simulink model "hbf_fft"  (R2015a)
settings: Solver=ode45  StartTime=0.0  StopTime=240300  RelTol=1e-3
model workspace (MAT data in the model file):
  MCOS : class17 (value not decoded)
  MCOS : class17 (value not decoded)
undefined symbols (not defined in the file or in its folder): a, b
libraries: xbsIndex_r4 x234, dspswit3 x1, commanapbnd3 x1, commseqgen2 x1, dspsigops x1
(part 2 of 2)

== system hbf_fft/nfftCounter/NegEdgeDet ==
  In1 : Inport
  Inverter : xbsIndex_r4/Inverter  en=off  latency=0  dbl_ovrd=off  block_type=inv
  Logical : xbsIndex_r4/Logical  logical_function=AND  inputs=2  en=off  latency=0  precision=Full  arith_type=Unsigned  n_bits=16  bin_pt=0  align_bp=on  dbl_ovrd=off  block_type=logical
  Register : xbsIndex_r4/Register  init=0  rst=off  en=off  dbl_ovrd=off  block_type=register
  Out1 : Outport
  wires:
  Register/1 -> Logical/1
  Inverter/1 -> Logical/2
  Logical/1 -> Out1/1
  In1/1 -> Inverter/1, Register/1

== system hbf_fft/nfftCounter/PosEdgeDet1 ==
  In1 : Inport
  Inverter : xbsIndex_r4/Inverter  en=off  latency=0  dbl_ovrd=off  block_type=inv
  Logical : xbsIndex_r4/Logical  logical_function=AND  inputs=2  en=off  latency=0  precision=Full  arith_type=Unsigned  n_bits=16  bin_pt=0  align_bp=on  dbl_ovrd=off  block_type=logical
  Register : xbsIndex_r4/Register  init=0  rst=off  en=off  dbl_ovrd=off  block_type=register
  Out1 : Outport
  wires:
  Logical/1 -> Out1/1
  In1/1 -> Logical/2, Register/1
  Register/1 -> Inverter/1
  Inverter/1 -> Logical/1

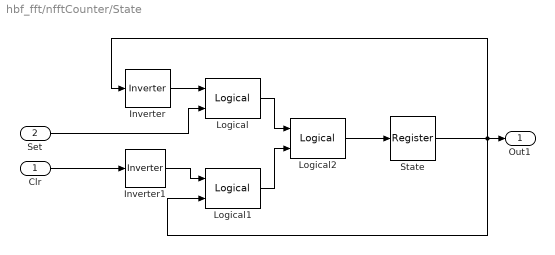
== system hbf_fft/nfftCounter/State ==
  Clr : Inport
  Set : Inport  Port=2
  Inverter : xbsIndex_r4/Inverter  en=off  latency=0  dbl_ovrd=off  block_type=inv
  Inverter1 : xbsIndex_r4/Inverter  en=off  latency=0  dbl_ovrd=off  block_type=inv
  Logical : xbsIndex_r4/Logical  logical_function=AND  inputs=2  en=off  latency=0  precision=Full  arith_type=Unsigned  n_bits=16  bin_pt=0  align_bp=on  dbl_ovrd=off  block_type=logical
  Logical1 : xbsIndex_r4/Logical  logical_function=AND  inputs=2  en=off  latency=0  precision=Full  arith_type=Unsigned  n_bits=16  bin_pt=0  align_bp=on  dbl_ovrd=off  block_type=logical
  Logical2 : xbsIndex_r4/Logical  logical_function=OR  inputs=2  en=off  latency=0  precision=Full  arith_type=Unsigned  n_bits=16  bin_pt=0  align_bp=on  dbl_ovrd=off  block_type=logical
  State : xbsIndex_r4/Register  init=0  rst=off  en=off  dbl_ovrd=off  block_type=register
  Out1 : Outport
  wires:
  Inverter1/1 -> Logical1/1
  Logical2/1 -> State/1
  Logical/1 -> Logical2/1
  Clr/1 -> Inverter1/1
  State/1 -> Out1/1, Logical1/2, Inverter/1
  Set/1 -> Logical/2
  Logical1/1 -> Logical2/2
  Inverter/1 -> Logical/1

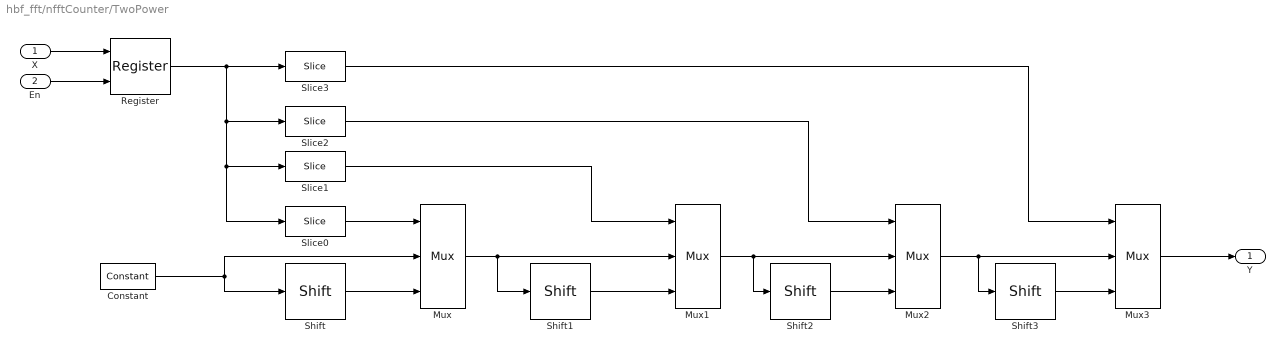
== system hbf_fft/nfftCounter/TwoPower ==
  X : Inport
  En : Inport  Port=2
  Constant : xbsIndex_r4/Constant  const=1.0  gui_display_data_type=Fixed-point  arith_type=Unsigned  n_bits=13  bin_pt=0  preci_type=Single  exp_width=8  frac_width=24  explicit_period=off  period=1  equ=P=C  opselect=C  inp2=PCIN>>17  opr=+  inp1=P  carry=CIN  dbl_ovrd=off  block_type=constant
  Mux : xbsIndex_r4/Mux  inputs=2  en=off  latency=0  precision=Full  arith_type=Unsigned  n_bits=16  bin_pt=14  quantization=Truncate  overflow=Wrap  dbl_ovrd=off  block_type=mux
  Mux1 : xbsIndex_r4/Mux  inputs=2  en=off  latency=0  precision=Full  arith_type=Unsigned  n_bits=16  bin_pt=14  quantization=Truncate  overflow=Wrap  dbl_ovrd=off  block_type=mux
  Mux2 : xbsIndex_r4/Mux  inputs=2  en=off  latency=0  precision=Full  arith_type=Unsigned  n_bits=16  bin_pt=14  quantization=Truncate  overflow=Wrap  dbl_ovrd=off  block_type=mux
  Mux3 : xbsIndex_r4/Mux  inputs=2  en=off  latency=1  precision=Full  arith_type=Unsigned  n_bits=16  bin_pt=14  quantization=Truncate  overflow=Wrap  dbl_ovrd=off  block_type=mux
  Register : xbsIndex_r4/Register  init=0  rst=off  en=on  dbl_ovrd=off  block_type=register
  Shift : xbsIndex_r4/Shift  shift_dir=Left  shift_bits=1  en=off  latency=0  precision=Full  arith_type="Signed  (2's comp)"  n_bits=16  bin_pt=14  quantization=Truncate  overflow=Wrap  dbl_ovrd=off  block_type=shift
  Shift1 : xbsIndex_r4/Shift  shift_dir=Left  shift_bits=2  en=off  latency=0  precision=Full  arith_type="Signed  (2's comp)"  n_bits=16  bin_pt=14  quantization=Truncate  overflow=Wrap  dbl_ovrd=off  block_type=shift
  Shift2 : xbsIndex_r4/Shift  shift_dir=Left  shift_bits=4  en=off  latency=0  precision=Full  arith_type="Signed  (2's comp)"  n_bits=16  bin_pt=14  quantization=Truncate  overflow=Wrap  dbl_ovrd=off  block_type=shift
  Shift3 : xbsIndex_r4/Shift  shift_dir=Left  shift_bits=8  en=off  latency=0  precision=Full  arith_type="Signed  (2's comp)"  n_bits=16  bin_pt=14  quantization=Truncate  overflow=Wrap  dbl_ovrd=off  block_type=shift
  Slice0 : xbsIndex_r4/Slice  nbits=1  boolean_output=off  mode=Lower Bit Location + Width  bit1=0  base1=MSB of Input  bit0=0  base0=LSB of Input  dbl_ovrd=off  block_type=slice
  Slice1 : xbsIndex_r4/Slice  nbits=1  boolean_output=off  mode=Lower Bit Location + Width  bit1=0  base1=MSB of Input  bit0=1  base0=LSB of Input  dbl_ovrd=off  block_type=slice
  Slice2 : xbsIndex_r4/Slice  nbits=1  boolean_output=off  mode=Lower Bit Location + Width  bit1=0  base1=MSB of Input  bit0=2  base0=LSB of Input  dbl_ovrd=off  block_type=slice
  Slice3 : xbsIndex_r4/Slice  nbits=1  boolean_output=off  mode=Lower Bit Location + Width  bit1=0  base1=MSB of Input  bit0=3  base0=LSB of Input  dbl_ovrd=off  block_type=slice
  Y : Outport
  wires:
  Constant/1 -> Shift/1, Mux/2
  X/1 -> Register/1
  Slice0/1 -> Mux/1
  Shift/1 -> Mux/3
  Slice1/1 -> Mux1/1
  Shift1/1 -> Mux1/3
  Slice2/1 -> Mux2/1
  Shift2/1 -> Mux2/3
  Slice3/1 -> Mux3/1
  Shift3/1 -> Mux3/3
  Mux/1 -> Shift1/1, Mux1/2
  Mux1/1 -> Shift2/1, Mux2/2
  Mux2/1 -> Shift3/1, Mux3/2
  Register/1 -> Slice0/1, Slice1/1, Slice2/1, Slice3/1
  En/1 -> Register/2
  Mux3/1 -> Y/1

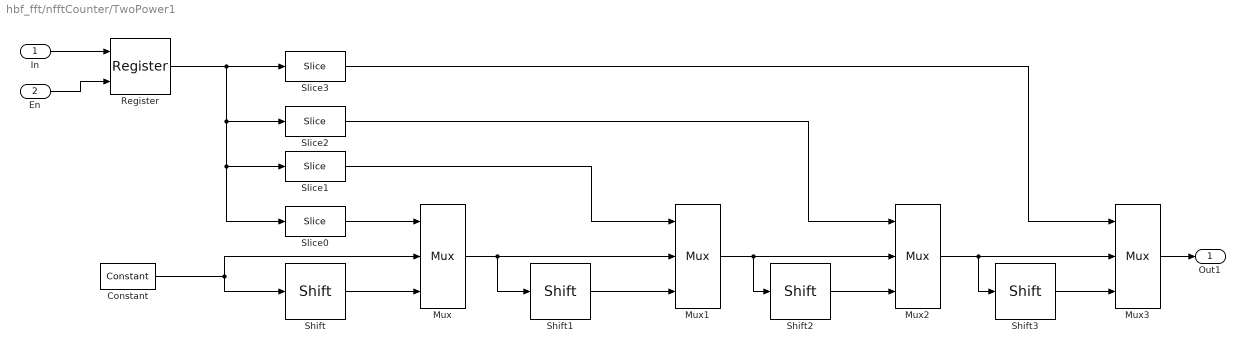
== system hbf_fft/nfftCounter/TwoPower1 ==
  In : Inport
  En : Inport  Port=2
  Constant : xbsIndex_r4/Constant  const=1.0  gui_display_data_type=Fixed-point  arith_type=Unsigned  n_bits=13  bin_pt=0  preci_type=Single  exp_width=8  frac_width=24  explicit_period=off  period=1  equ=P=C  opselect=C  inp2=PCIN>>17  opr=+  inp1=P  carry=CIN  dbl_ovrd=off  block_type=constant
  Mux : xbsIndex_r4/Mux  inputs=2  en=off  latency=0  precision=Full  arith_type=Unsigned  n_bits=16  bin_pt=14  quantization=Truncate  overflow=Wrap  dbl_ovrd=off  block_type=mux
  Mux1 : xbsIndex_r4/Mux  inputs=2  en=off  latency=0  precision=Full  arith_type=Unsigned  n_bits=16  bin_pt=14  quantization=Truncate  overflow=Wrap  dbl_ovrd=off  block_type=mux
  Mux2 : xbsIndex_r4/Mux  inputs=2  en=off  latency=0  precision=Full  arith_type=Unsigned  n_bits=16  bin_pt=14  quantization=Truncate  overflow=Wrap  dbl_ovrd=off  block_type=mux
  Mux3 : xbsIndex_r4/Mux  inputs=2  en=off  latency=1  precision=Full  arith_type=Unsigned  n_bits=16  bin_pt=14  quantization=Truncate  overflow=Wrap  dbl_ovrd=off  block_type=mux
  Register : xbsIndex_r4/Register  init=0  rst=off  en=on  dbl_ovrd=off  block_type=register
  Shift : xbsIndex_r4/Shift  shift_dir=Left  shift_bits=1  en=off  latency=0  precision=Full  arith_type="Signed  (2's comp)"  n_bits=16  bin_pt=14  quantization=Truncate  overflow=Wrap  dbl_ovrd=off  block_type=shift
  Shift1 : xbsIndex_r4/Shift  shift_dir=Left  shift_bits=2  en=off  latency=0  precision=Full  arith_type="Signed  (2's comp)"  n_bits=16  bin_pt=14  quantization=Truncate  overflow=Wrap  dbl_ovrd=off  block_type=shift
  Shift2 : xbsIndex_r4/Shift  shift_dir=Left  shift_bits=4  en=off  latency=0  precision=Full  arith_type="Signed  (2's comp)"  n_bits=16  bin_pt=14  quantization=Truncate  overflow=Wrap  dbl_ovrd=off  block_type=shift
  Shift3 : xbsIndex_r4/Shift  shift_dir=Left  shift_bits=8  en=off  latency=0  precision=Full  arith_type="Signed  (2's comp)"  n_bits=16  bin_pt=14  quantization=Truncate  overflow=Wrap  dbl_ovrd=off  block_type=shift
  Slice0 : xbsIndex_r4/Slice  nbits=1  boolean_output=off  mode=Lower Bit Location + Width  bit1=0  base1=MSB of Input  bit0=0  base0=LSB of Input  dbl_ovrd=off  block_type=slice
  Slice1 : xbsIndex_r4/Slice  nbits=1  boolean_output=off  mode=Lower Bit Location + Width  bit1=0  base1=MSB of Input  bit0=1  base0=LSB of Input  dbl_ovrd=off  block_type=slice
  Slice2 : xbsIndex_r4/Slice  nbits=1  boolean_output=off  mode=Lower Bit Location + Width  bit1=0  base1=MSB of Input  bit0=2  base0=LSB of Input  dbl_ovrd=off  block_type=slice
  Slice3 : xbsIndex_r4/Slice  nbits=1  boolean_output=off  mode=Lower Bit Location + Width  bit1=0  base1=MSB of Input  bit0=3  base0=LSB of Input  dbl_ovrd=off  block_type=slice
  Out1 : Outport
  wires:
  Constant/1 -> Shift/1, Mux/2
  In/1 -> Register/1
  Slice0/1 -> Mux/1
  Shift/1 -> Mux/3
  Slice1/1 -> Mux1/1
  Shift1/1 -> Mux1/3
  Slice2/1 -> Mux2/1
  Shift2/1 -> Mux2/3
  Slice3/1 -> Mux3/1
  Shift3/1 -> Mux3/3
  Mux/1 -> Shift1/1, Mux1/2
  Mux1/1 -> Shift2/1, Mux2/2
  Mux2/1 -> Shift3/1, Mux3/2
  Register/1 -> Slice0/1, Slice1/1, Slice2/1, Slice3/1
  En/1 -> Register/2
  Mux3/1 -> Out1/1

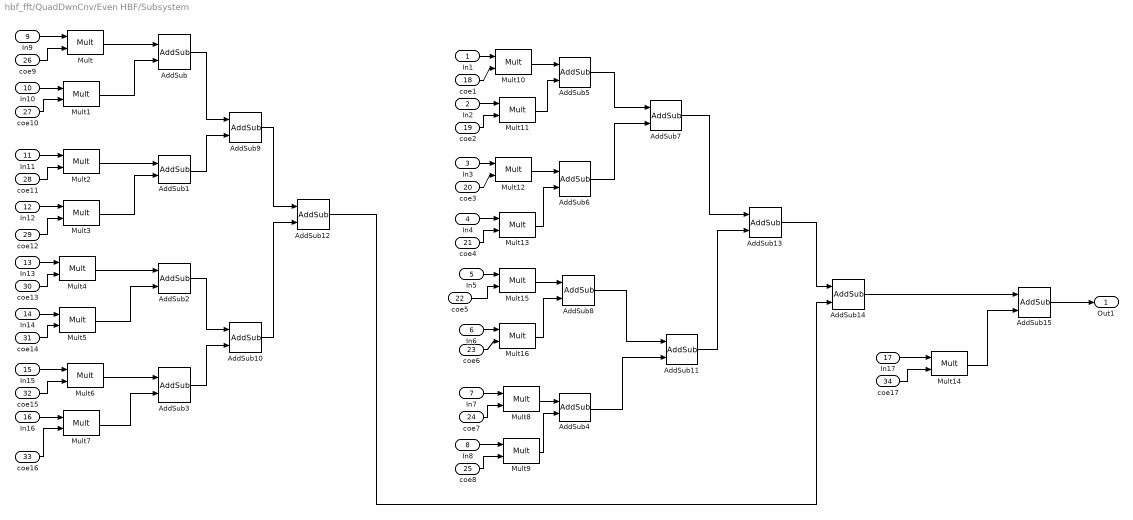
== system hbf_fft/QuadDwnCnv/Even HBF/Subsystem ==
  In1 : Inport
  In2 : Inport  Port=2
  In3 : Inport  Port=3
  In4 : Inport  Port=4
  In5 : Inport  Port=5
  In6 : Inport  Port=6
  In7 : Inport  Port=7
  In8 : Inport  Port=8
  In9 : Inport  Port=9
  In10 : Inport  Port=10
  In11 : Inport  Port=11
  In12 : Inport  Port=12
  In13 : Inport  Port=13
  In14 : Inport  Port=14
  In15 : Inport  Port=15
  In16 : Inport  Port=16
  In17 : Inport  Port=17
  coe1 : Inport  Port=18
  coe2 : Inport  Port=19
  coe3 : Inport  Port=20
  coe4 : Inport  Port=21
  coe5 : Inport  Port=22
  coe6 : Inport  Port=23
  coe7 : Inport  Port=24
  coe8 : Inport  Port=25
  coe9 : Inport  Port=26
  coe10 : Inport  Port=27
  coe11 : Inport  Port=28
  coe12 : Inport  Port=29
  coe13 : Inport  Port=30
  coe14 : Inport  Port=31
  coe15 : Inport  Port=32
  coe16 : Inport  Port=33
  coe17 : Inport  Port=34
  AddSub{,1..15} (16 alike) : xbsIndex_r4/AddSub  mode=Addition  use_carryin=off  use_carryout=off  en=off  latency=0  precision=Full  arith_type=Unsigned  n_bits=16  bin_pt=14  quantization=Truncate  overflow=Wrap  use_behavioral_HDL=off  hw_selection=Fabric  pipelined=off  use_rpm=on  dbl_ovrd=off  block_type=addsub
      settings: block_version=10.1.3
  Mult{,1..16} (17 alike) : xbsIndex_r4/Mult  precision=Full  arith_type="Signed  (2's comp)"  n_bits=16  bin_pt=14  quantization=Truncate  overflow=Wrap  en=off  latency=3  use_behavioral_HDL=off  opt=Speed  use_embedded=on  optimum_pipeline=off  pipeline=on  dbl_ovrd=off  use_rpm=on  placement_style=Triangular  block_type=mult
      settings: infoedit=Hardware notes: To use the internal pipeline stage of the dedicated multiplier you must select 'Pipeline for maximum performance'.  block_version=10.1.3
  Out1 : Outport
  wires:
  Mult/1 -> AddSub/1
  Mult1/1 -> AddSub/2
  Mult2/1 -> AddSub1/1
  Mult3/1 -> AddSub1/2
  Mult4/1 -> AddSub2/1
  Mult5/1 -> AddSub2/2
  Mult6/1 -> AddSub3/1
  Mult7/1 -> AddSub3/2
  Mult8/1 -> AddSub4/1
  Mult9/1 -> AddSub4/2
  Mult10/1 -> AddSub5/1
  Mult11/1 -> AddSub5/2
  Mult12/1 -> AddSub6/1
  Mult13/1 -> AddSub6/2
  Mult15/1 -> AddSub8/1
  In1/1 -> Mult10/1
  In2/1 -> Mult11/1
  In3/1 -> Mult12/1
  In4/1 -> Mult13/1
  In5/1 -> Mult15/1
  In6/1 -> Mult16/1
  In7/1 -> Mult8/1
  In8/1 -> Mult9/1
  In9/1 -> Mult/1
  In10/1 -> Mult1/1
  In11/1 -> Mult2/1
  In12/1 -> Mult3/1
  In13/1 -> Mult4/1
  In14/1 -> Mult5/1
  In15/1 -> Mult6/1
  In16/1 -> Mult7/1
  coe1/1 -> Mult10/2
  coe2/1 -> Mult11/2
  coe3/1 -> Mult12/2
  coe4/1 -> Mult13/2
  coe5/1 -> Mult15/2
  coe6/1 -> Mult16/2
  coe7/1 -> Mult8/2
  coe8/1 -> Mult9/2
  coe9/1 -> Mult/2
  coe10/1 -> Mult1/2
  coe11/1 -> Mult2/2
  coe12/1 -> Mult3/2
  coe13/1 -> Mult4/2
  coe14/1 -> Mult5/2
  coe15/1 -> Mult6/2
  coe16/1 -> Mult7/2
  In17/1 -> Mult14/1
  coe17/1 -> Mult14/2
  AddSub/1 -> AddSub9/1
  AddSub1/1 -> AddSub9/2
  AddSub2/1 -> AddSub10/1
  AddSub3/1 -> AddSub10/2
  AddSub5/1 -> AddSub7/1
  AddSub6/1 -> AddSub7/2
  AddSub8/1 -> AddSub11/1
  AddSub4/1 -> AddSub11/2
  AddSub9/1 -> AddSub12/1
  AddSub10/1 -> AddSub12/2
  AddSub7/1 -> AddSub13/1
  AddSub11/1 -> AddSub13/2
  AddSub13/1 -> AddSub14/1
  AddSub12/1 -> AddSub14/2
  AddSub14/1 -> AddSub15/1
  Mult14/1 -> AddSub15/2
  AddSub15/1 -> Out1/1
  Mult16/1 -> AddSub8/2
